simulink model "system_simulation_with_observer"  (R2024a)
settings: Solver=VariableStepAuto  StartTime=0.0  StopTime=2  RelTol=1e-3
values from neighbouring files (symbols this model uses):
  sys_init = randn(4, 1)    [sim_vars.m]
undefined symbols (not defined in the file or in its folder): A, B, C, F, FI, L
settings Model: Creator=balder  LastModifiedBy=balder

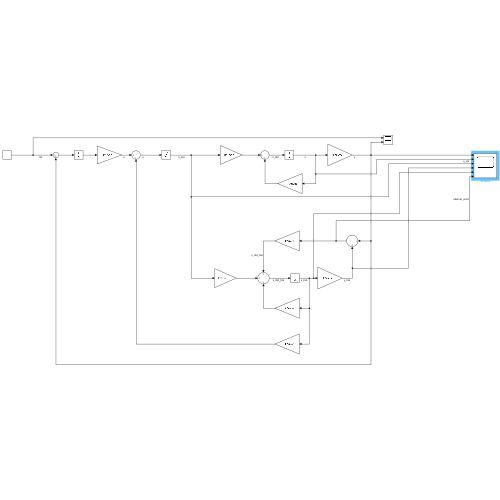
[thumbnail: Simulink's stored preview of the top-level diagram]
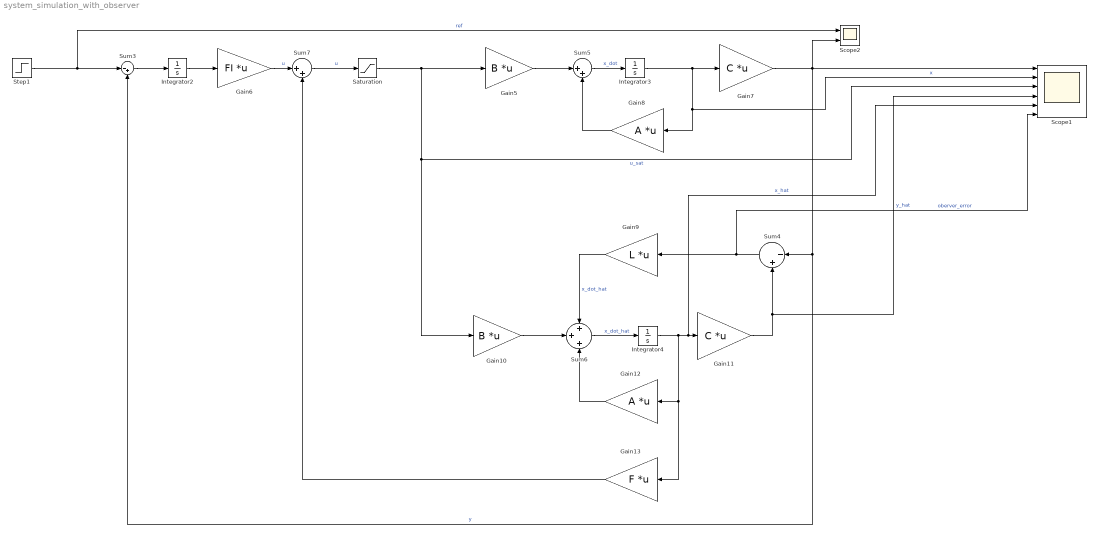
== system system_simulation_with_observer ==
  Gain10 : Gain  Gain=B  Multiplication=Matrix(K*u) (u vector)
  Gain11 : Gain  Gain=C  Multiplication=Matrix(K*u) (u vector)
  Gain12 : Gain  Gain=A  Multiplication=Matrix(K*u) (u vector)
  Gain13 : Gain  Gain=F  Multiplication=Matrix(K*u) (u vector)
  Gain5 : Gain  Gain=B  Multiplication=Matrix(K*u) (u vector)
  Gain6 : Gain  Gain=FI  Multiplication=Matrix(K*u) (u vector)
  Gain7 : Gain  Gain=C  Multiplication=Matrix(K*u) (u vector)
  Gain8 : Gain  Gain=A  Multiplication=Matrix(K*u) (u vector)
  Gain9 : Gain  Gain=L  Multiplication=Matrix(K*u) (u vector)
  Integrator2 : Integrator
  Integrator3 : Integrator  InitialCondition=sys_init
  Integrator4 : Integrator  UpperSaturationLimit=100  LowerSaturationLimit=-100
  Saturation : Saturate  UpperLimit=12  LowerLimit=-12
  Scope1 : Scope  NumInputPorts=6
  Scope2 : Scope  NumInputPorts=2
  Step1 : Step  Before=[0 0]  After=[1 -1]  SampleTime=0
  Sum3 : Sum  Inputs=|-+
  Sum4 : Sum  Inputs=|-+
  Sum5 : Sum  Inputs=|++
  Sum6 : Sum  Inputs=+++
  Sum7 : Sum  Inputs=|++
  wires:
  Sum5/1 -> Integrator3/1  "x_dot"
  Gain7/1 -> Scope2/2, Scope1/1, Sum4/1, Sum3/2  "y"
  Integrator4/1 -> Gain11/1, Scope1/5, Gain13/1, Gain12/1  "x_hat"
  Sum7/1 -> Saturation/1  "u"
  Gain5/1 -> Sum5/1
  Saturation/1 -> Gain5/1, Gain10/1, Scope1/3  "u_sat"
  Sum3/1 -> Integrator2/1
  Gain11/1 -> Scope1/4, Sum4/2  "y_hat"
  Sum6/1 -> Integrator4/1  "x_dot_hat"
  Integrator2/1 -> Gain6/1
  Gain9/1 -> Sum6/1  "x_dot_hat"
  Sum4/1 -> Scope1/6, Gain9/1  "oberver_error"
  Step1/1 -> Scope2/1, Sum3/1  "ref"
  Gain6/1 -> Sum7/1  "u"
  Integrator3/1 -> Gain8/1, Scope1/2, Gain7/1  "x"
  Gain13/1 -> Sum7/2
  Gain10/1 -> Sum6/2
  Gain12/1 -> Sum6/3
  Gain8/1 -> Sum5/2
